simulink model "position_to_velocity_controller"  (R2017a)
settings: Solver=VariableStepAuto  StartTime=0.0  StopTime=10.0  RelTol=1e-3
undefined symbols (not defined in the file or in its folder): antiwindup
settings Model: Creator=maxwell  LastModifiedBy=maxwell

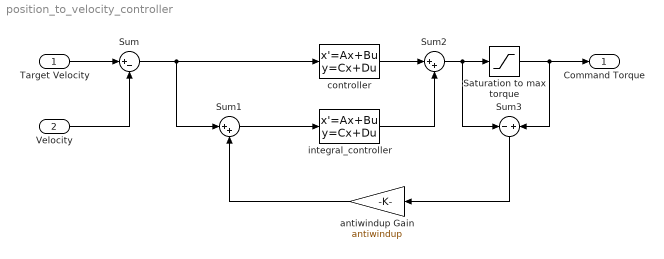
== system position_to_velocity_controller ==
  Target Velocity : Inport
  Velocity : Inport  Port=2
  Saturation to max torque : Saturate
  Sum : Sum  Inputs=|+-
  Sum1 : Sum  Inputs=|++
  Sum2 : Sum  Inputs=|++
  Sum3 : Sum  Inputs=-+
  antiwindup Gain : Gain  Gain=antiwindup
  controller : StateSpace  X0=0
  integral_controller : StateSpace  X0=0
  Command Torque : Outport
  wires:
  Sum/1 -> Sum1/1, controller/1
  Sum1/1 -> integral_controller/1
  controller/1 -> Sum2/1
  integral_controller/1 -> Sum2/2
  Sum2/1 -> Sum3/1, Saturation to max torque/1
  Saturation to max torque/1 -> Command Torque/1, Sum3/2
  Sum3/1 -> antiwindup Gain/1
  antiwindup Gain/1 -> Sum1/2
  Target Velocity/1 -> Sum/1
  Velocity/1 -> Sum/2
